simulink model "FingerStrokeAssistance"  (R2016a)
settings: Solver=FixedStepDiscrete  StartTime=0.0  StopTime=inf  FixedStep=.001  RelTol=1e-3
PreLoadFcn:
  | settupFilter;
InitFcn:
  | settupFilter;
  | xpctargetping
values from neighbouring files (symbols this model uses):
  x0low = (eye(size(Alow))-Alow)\Blow*0    [settupFilter.m]
undefined symbols (not defined in the file or in its folder): a_hp, a_lp, Alow, b_hp, b_lp, Blow, Clow, DiscIntNeverNeededParam, Dlow
libraries: simulink x8, slrtlib x8, xpcnilib x4
settings Model: SimulationMode=external  Creator=Admin  LastModifiedBy=Juno
settings SolverCC: EnableConcurrentExecution=on
settings DataIOCC: LimitDataPoints=on  SaveFormat=Array
settings OptimizationCC: BlockReduction=off  OptimizeBlockIOStorage=off  BufferReuse=off  GlobalBufferReuse=off  ExpressionFolding=off  ExpressionDepthLimit=2147483647  LocalBlockOutputs=off
settings DebuggingCC: UnderspecifiedInitializationDetection=Classic  MergeDetectMultiDrivingBlocksExec=none  SolverPrmCheckMsg=warning  StateNameClashWarn=warning
settings HardwareCC: ProdBitPerPointer=32  ProdLargestAtomicFloat=None  ProdWordSize=32  ProdLongLongMode=on  ProdHWDeviceType=Generic->32-bit x86 compatible
settings ModelReferenceCC: PropagateSignalLabelsOutOfModel=off
settings RTWCC: SystemTargetFile=slrt.tlc  TemplateMakefile=slrt_default_tmf  Description=Simulink Real-Time  RTWCompilerOptimization=on
settings ConfigComp: CovModelRefEnable=Off

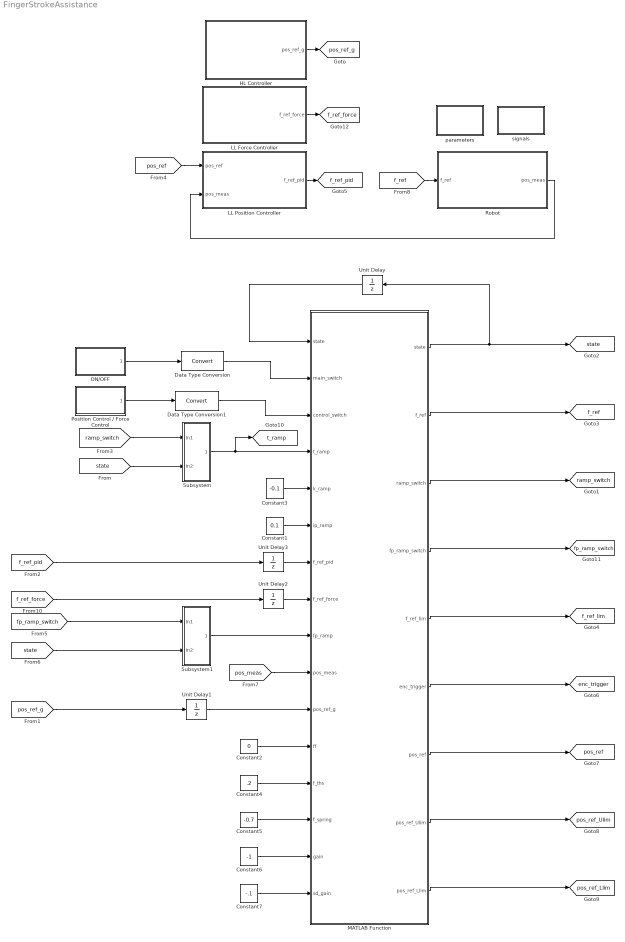
== system FingerStrokeAssistance ==
  Constant1 : Constant  Value=0.1
  Constant2 : Constant  Value=0
  Constant3 : Constant  Value=-0.1
  Constant4 : Constant  Value=.2
  Constant5 : Constant  Value=-0.7
  Constant6 : Constant  Value=-1
  Constant7 : Constant  Value=-.1
  Data Type Conversion : DataTypeConversion
  Data Type Conversion1 : DataTypeConversion
  HL Controller : Subsystem
  LL Force Controller : Subsystem
  LL Position Controller : Subsystem
  MATLAB Function : MATLAB Function  TreatAsAtomicUnit=on
      settings: MinAlgLoopOccurrences=on
  ON/OFF : Subsystem  InitFcn=|  StartFcn=|  StopFcn=|
      InitFcn=|
      | set_param([gcb,'/Constant'],'value','0');                    
      | set_param(gcb,'BackgroundColor',sprintf('[%f,%f,%f]',1,0,0));
      |                                                              
      | set_param(gcb,'MaskDisplay', ['disp(''Not Running'')']);
      StartFcn=|
      | set_param([gcb,'/Constant'],'value','0');                    
      | set_param(gcb,'BackgroundColor',sprintf('[%f,%f,%f]',1,0,0));
      |                                                              
      | set_param(gcb,'MaskDisplay', ['disp(''Not Running'')']);
      StopFcn=|
      | set_param([gcb,'/Constant'],'value','0');                    
      | set_param(gcb,'BackgroundColor',sprintf('[%f,%f,%f]',1,0,0));
      | set_param(gcb,'MaskDisplay', ['disp(''Not Running'')']);
      settings: OpenFcn=|
      | currentState = str2num(get_param([gcb,'/Constant'],'value'));
      | if currentState==1;                                                                       set_param([gcb,'/Constant'],'value','0');
      | set_param(gcb,'BackgroundColor',sprintf('[%f,%f,%f]',1,0,0));                                                   set_param(gcb,'MaskDisplay', ['disp(''Not Running'')']);
      | else                                                                                                                             set_param([gcb,'/Constant'],'value','1');
      | set_param(gcb,'BackgroundColor',sprintf('[%f,%f,%f]',0,1,0));                                            set_param(gcb,'MaskDisplay', ['disp(''Running'')']);
      | 
      | end
      mask Display: disp('Not Running')
  Position Control / Force Control : Subsystem  InitFcn=|  StartFcn=|  StopFcn=|
      InitFcn=|
      | set_param([gcb,'/Constant'],'value','0');                    
      | set_param(gcb,'BackgroundColor',sprintf('[%f,%f,%f]',1,0,0));
      |                                                              
      | set_param(gcb,'MaskDisplay', ['disp(''Not Running'')']);
      StartFcn=|
      | set_param([gcb,'/Constant'],'value','0');                    
      | set_param(gcb,'BackgroundColor',sprintf('[%f,%f,%f]',1,0,0));
      |                                                              
      | set_param(gcb,'MaskDisplay', ['disp(''Not Running'')']);
      StopFcn=|
      | set_param([gcb,'/Constant'],'value','0');                    
      | set_param(gcb,'BackgroundColor',sprintf('[%f,%f,%f]',1,0,0));
      | set_param(gcb,'MaskDisplay', ['disp(''Not Running'')']);
      settings: OpenFcn=|
      | currentState = str2num(get_param([gcb,'/Constant'],'value'));
      | if currentState==1;                                                                       set_param([gcb,'/Constant'],'value','0');
      | set_param(gcb,'BackgroundColor',sprintf('[%f,%f,%f]',1,0,0));                                                   set_param(gcb,'MaskDisplay', ['disp(''Not Running'')']);
      | else                                                                                                                             set_param([gcb,'/Constant'],'value','1');
      | set_param(gcb,'BackgroundColor',sprintf('[%f,%f,%f]',0,1,0));                                            set_param(gcb,'MaskDisplay', ['disp(''Running'')']);
      | 
      | end
      mask Display: disp('Not Running')
  Robot : Subsystem
  Subsystem : Subsystem
  Subsystem1 : Subsystem
  Unit Delay : UnitDelay  InitialCondition=1  SampleTime=-1
  Unit Delay1 : UnitDelay  SampleTime=-1
  Unit Delay2 : UnitDelay  SampleTime=-1
  Unit Delay3 : UnitDelay  SampleTime=-1
  parameters : Subsystem
  signals : Subsystem
  tag scope: enc_trigger=global, f_ref=global, f_ref_force=global, f_ref_lim=global, f_ref_pid=global, fp_ramp_switch=global, pos_ref=global, pos_ref_Llim=global, pos_ref_Ulim=global, pos_ref_g=global, ramp_switch=global, state=global, t_ramp=global
  wires:
  Robot/1(pos_meas) -> LL Position Controller/2(pos_meas)
  MATLAB Function/1(state) -> Unit Delay/1, [state]
  MATLAB Function/2(f_ref) -> [f_ref]
  Constant3/1 -> MATLAB Function/5(k_ramp)
  MATLAB Function/5(f_ref_lim) -> [f_ref_lim]
  MATLAB Function/3(ramp_switch) -> [ramp_switch]
  MATLAB Function/6(enc_trigger) -> [enc_trigger]
  Constant1/1 -> MATLAB Function/6(ip_ramp)
  [f_ref_pid] -> Unit Delay3/1
  MATLAB Function/8(pos_ref_Ulim) -> [pos_ref_Ulim]
  MATLAB Function/9(pos_ref_Llim) -> [pos_ref_Llim]
  [pos_ref] -> LL Position Controller/1(pos_ref)
  MATLAB Function/7(pos_ref) -> [pos_ref]
  Unit Delay3/1 -> MATLAB Function/7(f_ref_pid)
  Subsystem/1(Out1) -> [t_ramp], MATLAB Function/4(t_ramp)
  [ramp_switch] -> Subsystem/1(In1)
  [state] -> Subsystem/2(In2)
  [fp_ramp_switch] -> Subsystem1/1(In1)
  [state] -> Subsystem1/2(In2)
  MATLAB Function/4(fp_ramp_switch) -> [fp_ramp_switch]
  Subsystem1/1(Out1) -> MATLAB Function/9(fp_ramp)
  [pos_meas] -> MATLAB Function/10(pos_meas)
  ON/OFF/1(" ") -> Data Type Conversion/1
  Unit Delay/1 -> MATLAB Function/1("state ")
  [pos_ref_g] -> Unit Delay1/1
  Unit Delay1/1 -> MATLAB Function/11(pos_ref_g)
  LL Position Controller/1(" f_ref_pid") -> [f_ref_pid]
  [f_ref] -> Robot/1(f_ref)
  Data Type Conversion/1 -> MATLAB Function/2(main_switch)
  HL Controller/1(pos_ref_g) -> [pos_ref_g]
  Position Control / Force Control/1(" ") -> Data Type Conversion1/1
  Data Type Conversion1/1 -> MATLAB Function/3(control_switch)
  [f_ref_force] -> Unit Delay2/1
  Unit Delay2/1 -> MATLAB Function/8(f_ref_force)
  LL Force Controller/1(" f_ref_force") -> [f_ref_force]
  Constant2/1 -> MATLAB Function/12(ff)
  Constant5/1 -> MATLAB Function/14(f_spring)
  Constant6/1 -> MATLAB Function/15(gain)
  Constant4/1 -> MATLAB Function/13(f_ths)
  Constant7/1 -> MATLAB Function/16(sd_gain)

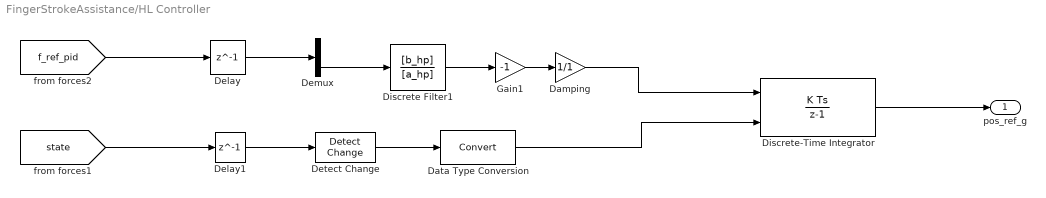
== system FingerStrokeAssistance/HL Controller ==
  Damping : Gain  Gain=1/1
  Data Type Conversion : DataTypeConversion
  Delay : Delay  DelayLength=1  InitialCondition=0
  Delay1 : Delay  DelayLength=1  InitialCondition=0
  Demux : Demux  Outputs=2
  Detect Change : simulink/Logic and Bit Operations/Detect Change  vinit=0  OutDataTypeStr=boolean
  Discrete Filter1 : DiscreteFilter  Numerator=[b_hp]  Denominator=[a_hp]
  Discrete-Time Integrator : DiscreteIntegrator  ExternalReset=either  InitialConditionSetting=State (most efficient)  SampleTime=-1  LimitOutput=on  UpperSaturationLimit=1  LowerSaturationLimit=0  ICPrevOutput=DiscIntNeverNeededParam  ICPrevScaledInput=DiscIntNeverNeededParam
  Gain1 : Gain  Gain=-1
  pos_ref_g : Outport
  wires:
  [f_ref_pid] -> Delay/1
  [state] -> Delay1/1
  Discrete-Time Integrator/1 -> pos_ref_g/1
  Detect Change/1 -> Data Type Conversion/1
  Delay1/1 -> Detect Change/1
  Delay/1 -> Demux/1
  Data Type Conversion/1 -> Discrete-Time Integrator/2
  Gain1/1 -> Damping/1
  Damping/1 -> Discrete-Time Integrator/1
  Demux/2 -> Discrete Filter1/1
  Discrete Filter1/1 -> Gain1/1

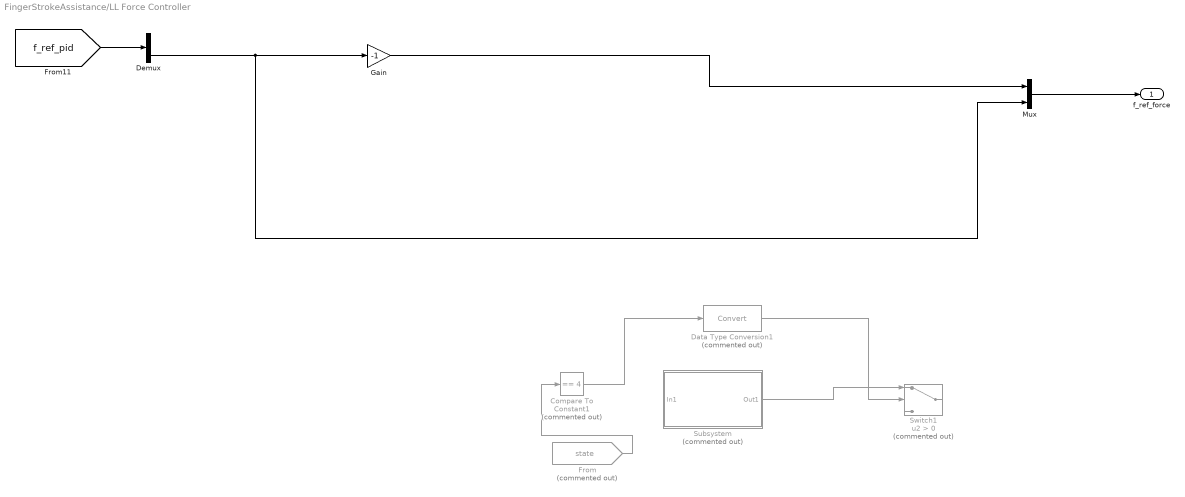
== system FingerStrokeAssistance/LL Force Controller ==
  Compare To Constant1 : simulink/Logic and Bit Operations/Compare To Constant  Commented=on  relop===  const=4  OutDataTypeStr=boolean
  Data Type Conversion1 : DataTypeConversion  Commented=on
  Demux : Demux  Outputs=2
  From : From  Commented=on  GotoTag=state  TagVisibility=global
  Gain : Gain  Gain=-1
  Mux : Mux  Inputs=2
  Subsystem : Subsystem  Commented=on
  Switch1 : Switch  Commented=on  Criteria=u2 > Threshold
  " f_ref_force" : Outport
  wires:
  [f_ref_pid] -> Demux/1
  Demux/2 -> Mux/2, Gain/1
  Subsystem/1(Out1) -> Switch1/1
  Data Type Conversion1/1 -> Switch1/2
  From/1 -> Compare To Constant1/1
  Compare To Constant1/1 -> Data Type Conversion1/1
  Mux/1 -> " f_ref_force"/1
  Gain/1 -> Mux/1

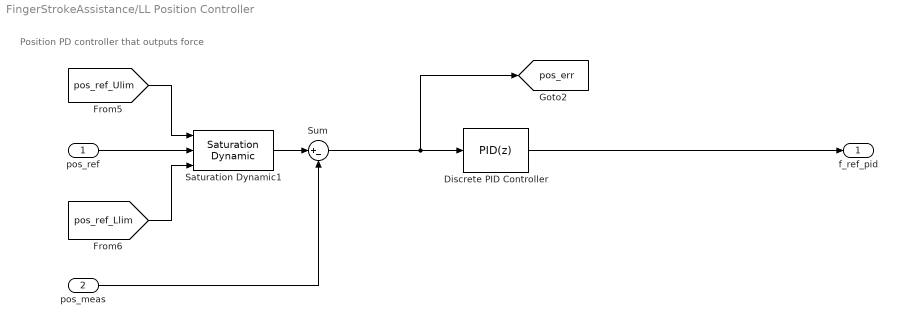
== system FingerStrokeAssistance/LL Position Controller ==
  note: Position PD controller that outputs force
  pos_ref : Inport
  pos_meas : Inport  Port=2
  Discrete PID Controller : simulink/Continuous/PID Controller  Controller=PID  TimeDomain=Discrete-time  SampleTime=-1  IntegratorMethod=Forward Euler  FilterMethod=Forward Euler  Form=Parallel  UseFilter=on  ControllerParametersSource=internal  P=10  I=0  D=0  N=100  InitialConditionSource=internal  InitialConditionForIntegrator=0  InitialConditionForFilter=0  ExternalReset=none  LimitOutput=off  UpperSaturationLimit=inf  LowerSaturationLimit=-inf  LinearizeAsGain=off  AntiWindupMode=none  Kb=1  TrackingMode=off  Kt=1  PParamMin=[]  PParamMax=[]  IParamMin=[]  IParamMax=[]  DParamMin=[]  DParamMax=[]  NParamMin=[]  NParamMax=[]  KbParamMin=[]  KbParamMax=[]  KtParamMin=[]  KtParamMax=[]  POutMin=[]  POutMax=[]  IOutMin=[]  IOutMax=[]  DOutMin=[]  DOutMax=[]  NOutMin=[]  NOutMax=[]  KbOutMin=[]  KbOutMax=[]  KtOutMin=[]  KtOutMax=[]  IntegratorOutMin=[]  IntegratorOutMax=[]  FilterOutMin=[]  FilterOutMax=[]  SumOutMin=[]  SumOutMax=[]  SumI1OutMin=[]  SumI1OutMax=[]  SumI2OutMin=[]  SumI2OutMax=[]  SumI3OutMin=[]  SumI3OutMax=[]  SumDOutMin=[]  SumDOutMax=[]  SaturationOutMin=[]  SaturationOutMax=[]  IntegratorContinuousStateAttributes=''  IntegratorStateMustResolveToSignalObject=off  IntegratorRTWStateStorageClass=Auto  FilterContinuousStateAttributes=''  FilterStateMustResolveToSignalObject=off  FilterRTWStateStorageClass=Auto  DifferentiatorICPrevScaledInput=0  DifferentiatorOutMin=[]  DifferentiatorOutMax=[]
  Saturation Dynamic1 : simulink/Discontinuities/Saturation Dynamic  OutMin=[]  OutMax=[]  OutDataTypeStr=Inherit: Same as second input  OutDataType=fixdt(1, 16)  OutScaling=2^-10  DoSatur=off
  Sum : Sum  Inputs=|+-
  " f_ref_pid" : Outport
  tag scope: pos_err=global
  wires:
  pos_meas/1 -> Sum/2
  Sum/1 -> Discrete PID Controller/1, [pos_err]
  Saturation Dynamic1/1 -> Sum/1
  pos_ref/1 -> Saturation Dynamic1/2
  [pos_ref_Ulim] -> Saturation Dynamic1/1
  [pos_ref_Llim] -> Saturation Dynamic1/3
  Discrete PID Controller/1 -> " f_ref_pid"/1

== system FingerStrokeAssistance/ON//OFF ==
  note: ON/OFF
  Constant : Constant  Value=0  OutDataTypeStr=boolean
  " " : Outport
  wires:
  Constant/1 -> " "/1

== system FingerStrokeAssistance/Position Control // Force Control ==
  note: ON/OFF
  Constant : Constant  Value=0  OutDataTypeStr=boolean
  " " : Outport
  wires:
  Constant/1 -> " "/1

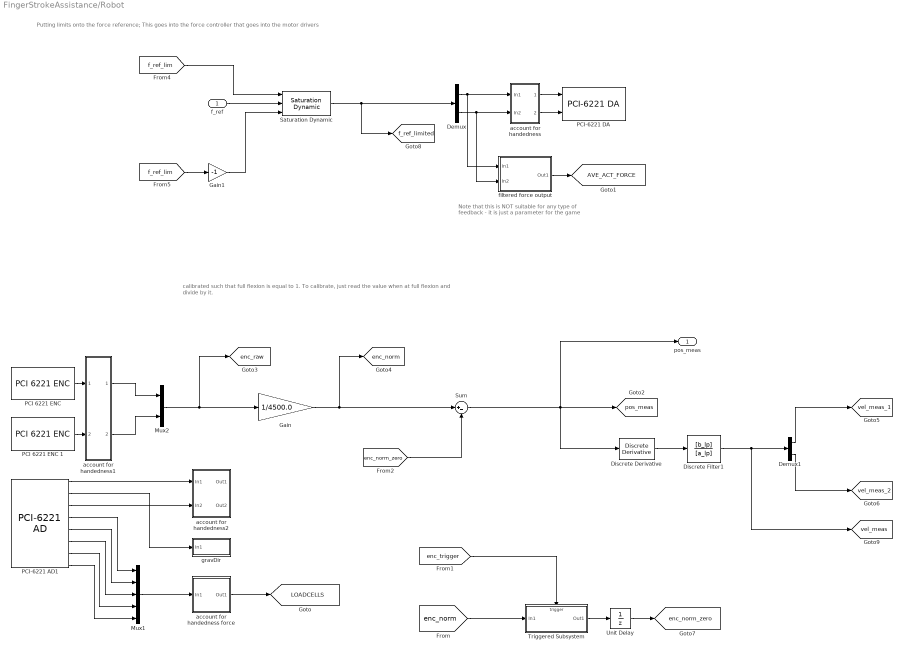
== system FingerStrokeAssistance/Robot ==
  note: Note that this is NOT suitable for any type
      | of feedback - it is just a parameter for the game
  note: calibrated such that full flexion is equal to 1. To calibrate, just read the value when at full flexion and divide by it.
  note: Putting limits onto the force reference; This goes into the force controller that goes into the motor drivers
  f_ref : Inport
  Demux : Demux  Outputs=2
  Demux1 : Demux  Outputs=2
  Discrete Derivative : simulink/Discrete/Discrete Derivative  gainval=1.0  ICPrevScaledInput=0.0  OutMin=[]  OutMax=[]  OutDataType=fixdt(1, 16)  OutScaling=2^-10  DoSatur=off
  Discrete Filter1 : DiscreteFilter  Numerator=[b_lp]  Denominator=[a_lp]
  Gain : Gain  Gain=1/4500.0
  Gain1 : Gain  Gain=-1
  Mux1 : Mux  Inputs=5
  Mux2 : Mux  Inputs=2
  "PCI 6221 ENC " : xpcnilib/Incremental Encoder/PCI 6221 ENC   channel=0  countMode=Quadrature Mode x4  initCount=0  reload=off  indexPhase=A low B low  filter=Minimum pulse width 125 nanoseconds  sampleTime=0.001  slot=-1
  PCI 6221 ENC 1 : xpcnilib/Incremental Encoder/PCI 6221 ENC   channel=1  countMode=Quadrature Mode x4  initCount=0  reload=off  indexPhase=A low B low  filter=Minimum pulse width 125 nanoseconds  sampleTime=0.001  slot=-1
  PCI-6221 AD1 : xpcnilib/A//D/M Series/PCI-6221 AD  channel=[1 2 3 4 5 6 7 8]  range=[10]  coupling=[0]  scantime=5e-6  sampletime=0.001  slot=-1
  PCI-6221 DA : xpcnilib/D//A/M Series/PCI-6221 DA  channel=[1 2]  reset=[1]  initValue=[0]  sampletime=0.001  slot=-1
  Saturation Dynamic : simulink/Discontinuities/Saturation Dynamic  OutMin=[]  OutMax=[]  OutDataTypeStr=Inherit: Same as second input  OutDataType=fixdt(1, 16)  OutScaling=2^-10  DoSatur=off
  Sum : Sum  Inputs=|+-
  Triggered Subsystem : Subsystem  TreatAsAtomicUnit=on
  Unit Delay : UnitDelay  SampleTime=-1
  account for handedness : Subsystem
  account for handedness force : Subsystem
  account for handedness1 : Subsystem
  account for handedness2 : Subsystem
  filtered force output : Subsystem
  gravDir : Subsystem
  pos_meas : Outport
  tag scope: AVE_ACT_FORCE=global, LOADCELLS=global, enc_norm=global, enc_norm_zero=global, enc_raw=global, f_ref_limited=global, pos_meas=global, vel_meas=global, vel_meas_1=global, vel_meas_2=global
  wires:
  Demux/1 -> filtered force output/1(In1), account for handedness/1(In1)
  Demux/2 -> filtered force output/2(In2), account for handedness/2(In2)
  account for handedness/2(Out2) -> PCI-6221 DA/2
  account for handedness/1(Out1) -> PCI-6221 DA/1
  "PCI 6221 ENC "/1 -> account for handedness1/1(In1)
  PCI 6221 ENC 1/1 -> account for handedness1/2(In2)
  PCI-6221 AD1/1 -> account for handedness2/1(In1)
  PCI-6221 AD1/3 -> account for handedness2/2(In2)
  PCI-6221 AD1/4 -> Mux1/1
  PCI-6221 AD1/5 -> Mux1/2
  PCI-6221 AD1/6 -> Mux1/3
  PCI-6221 AD1/7 -> Mux1/4
  PCI-6221 AD1/8 -> Mux1/5
  Mux1/1 -> account for handedness force/1(In1)
  account for handedness force/1(Out1) -> [LOADCELLS]
  PCI-6221 AD1/2 -> gravDir/1(In1)
  filtered force output/1(Out1) -> [AVE_ACT_FORCE]
  account for handedness1/1(Out1) -> Mux2/1
  account for handedness1/2(Out2) -> Mux2/2
  Mux2/1 -> [enc_raw], Gain/1
  Demux1/1 -> [vel_meas_1]
  Demux1/2 -> [vel_meas_2]
  Gain/1 -> Sum/1, [enc_norm]
  [enc_norm] -> Triggered Subsystem/1(In1)
  Triggered Subsystem/1(Out1) -> Unit Delay/1
  [enc_norm_zero] -> Sum/2
  Unit Delay/1 -> [enc_norm_zero]
  Sum/1 -> [pos_meas], pos_meas/1, Discrete Derivative/1
  [enc_trigger] -> Triggered Subsystem/Trigger
  Saturation Dynamic/1 -> [f_ref_limited], Demux/1
  Gain1/1 -> Saturation Dynamic/3
  [f_ref_lim] -> Saturation Dynamic/1
  [f_ref_lim] -> Gain1/1
  f_ref/1 -> Saturation Dynamic/2
  Discrete Derivative/1 -> Discrete Filter1/1
  Discrete Filter1/1 -> [vel_meas], Demux1/1

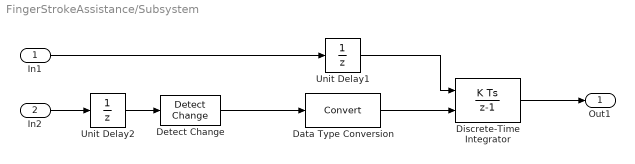
== system FingerStrokeAssistance/Subsystem ==
  In1 : Inport
  In2 : Inport  Port=2
  Data Type Conversion : DataTypeConversion
  Detect Change : simulink/Logic and Bit Operations/Detect Change  vinit=0  OutDataTypeStr=boolean
  Discrete-Time Integrator : DiscreteIntegrator  ExternalReset=either  InitialConditionSetting=State (most efficient)  SampleTime=-1  UpperSaturationLimit=0.9  LowerSaturationLimit=0  ICPrevOutput=DiscIntNeverNeededParam  ICPrevScaledInput=DiscIntNeverNeededParam
  Unit Delay1 : UnitDelay  SampleTime=-1
  Unit Delay2 : UnitDelay  SampleTime=-1
  Out1 : Outport
  wires:
  In1/1 -> Unit Delay1/1
  Unit Delay1/1 -> Discrete-Time Integrator/1
  Discrete-Time Integrator/1 -> Out1/1
  In2/1 -> Unit Delay2/1
  Data Type Conversion/1 -> Discrete-Time Integrator/2
  Detect Change/1 -> Data Type Conversion/1
  Unit Delay2/1 -> Detect Change/1

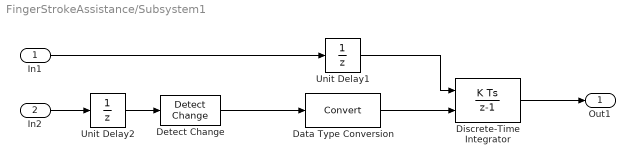
== system FingerStrokeAssistance/Subsystem1 ==
  In1 : Inport
  In2 : Inport  Port=2
  Data Type Conversion : DataTypeConversion
  Detect Change : simulink/Logic and Bit Operations/Detect Change  vinit=0  OutDataTypeStr=boolean
  Discrete-Time Integrator : DiscreteIntegrator  ExternalReset=either  InitialConditionSetting=State (most efficient)  SampleTime=-1  UpperSaturationLimit=0.9  LowerSaturationLimit=0  ICPrevOutput=DiscIntNeverNeededParam  ICPrevScaledInput=DiscIntNeverNeededParam
  Unit Delay1 : UnitDelay  SampleTime=-1
  Unit Delay2 : UnitDelay  SampleTime=-1
  Out1 : Outport
  wires:
  Unit Delay2/1 -> Detect Change/1
  Detect Change/1 -> Data Type Conversion/1
  Data Type Conversion/1 -> Discrete-Time Integrator/2
  In2/1 -> Unit Delay2/1
  Discrete-Time Integrator/1 -> Out1/1
  Unit Delay1/1 -> Discrete-Time Integrator/1
  In1/1 -> Unit Delay1/1

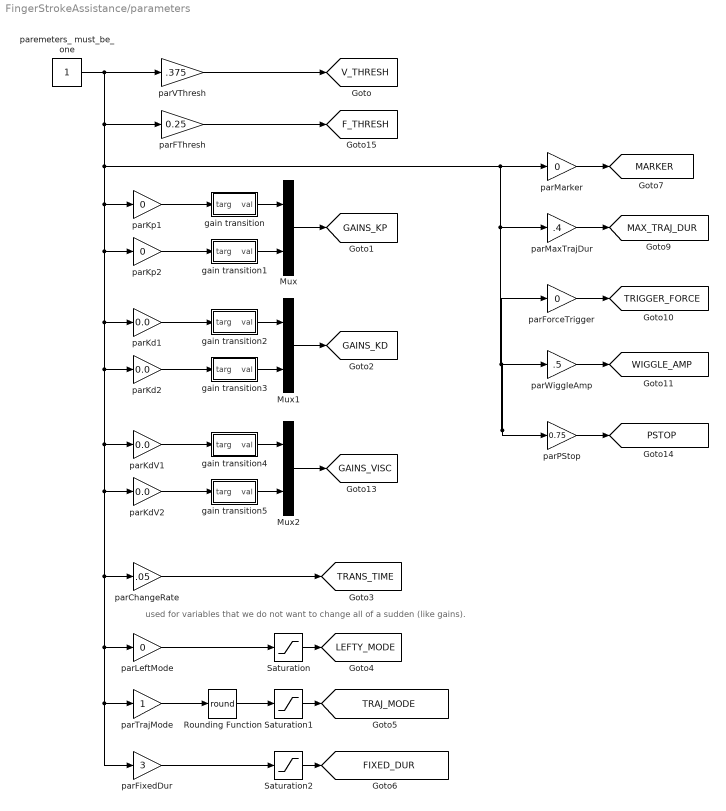
== system FingerStrokeAssistance/parameters ==
  note: used for variables that we do not want to change all of a sudden (like gains).
  Mux : Mux  Inputs=2
  Mux1 : Mux  Inputs=2
  Mux2 : Mux  Inputs=2
  Rounding Function : Rounding  Operator=round
  Saturation : Saturate  UpperLimit=1  LowerLimit=0
  Saturation1 : Saturate  UpperLimit=4  LowerLimit=1
  Saturation2 : Saturate  UpperLimit=10  LowerLimit=.25
  gain transition : Subsystem
  gain transition1 : Subsystem
  gain transition2 : Subsystem
  gain transition3 : Subsystem
  gain transition4 : Subsystem
  gain transition5 : Subsystem
  parChangeRate : Gain  Gain=.05
  parFThresh : Gain  Gain=0.25
  parFixedDur : Gain  Gain=3
  parForceTrigger : Gain  Gain=0
  parKd1 : Gain  Gain=0.0
  parKd2 : Gain  Gain=0.0
  parKdV1 : Gain  Gain=0.0
  parKdV2 : Gain  Gain=0.0
  parKp1 : Gain  Gain=0
  parKp2 : Gain  Gain=0
  parLeftMode : Gain  Gain=0
  parMarker : Gain  Gain=0
  parMaxTrajDur : Gain  Gain=.4
  parPStop : Gain  Gain=0.75
  parTrajMode : Gain
  parVThresh : Gain  Gain=.375
  parWiggleAmp : Gain  Gain=.5
  paremeters_ must_be_one : Constant
  tag scope: FIXED_DUR=global, F_THRESH=global, GAINS_KD=global, GAINS_KP=global, GAINS_VISC=global, LEFTY_MODE=global, MARKER=global, MAX_TRAJ_DUR=global, PSTOP=global, TRAJ_MODE=global, TRANS_TIME=global, TRIGGER_FORCE=global, V_THRESH=global, WIGGLE_AMP=global
  wires:
  Mux/1 -> [GAINS_KP]
  Mux1/1 -> [GAINS_KD]
  Saturation/1 -> [LEFTY_MODE]
  gain transition/1(val) -> Mux/1
  gain transition1/1(val) -> Mux/2
  gain transition2/1(val) -> Mux1/1
  gain transition3/1(val) -> Mux1/2
  parVThresh/1 -> [V_THRESH]
  parKp1/1 -> gain transition/1(targ)
  parKp2/1 -> gain transition1/1(targ)
  parKd1/1 -> gain transition2/1(targ)
  parKd2/1 -> gain transition3/1(targ)
  parChangeRate/1 -> [TRANS_TIME]
  parLeftMode/1 -> Saturation/1
  Saturation1/1 -> [TRAJ_MODE]
  parTrajMode/1 -> Rounding Function/1
  Saturation2/1 -> [FIXED_DUR]
  parFixedDur/1 -> Saturation2/1
  Rounding Function/1 -> Saturation1/1
  parMarker/1 -> [MARKER]
  parMaxTrajDur/1 -> [MAX_TRAJ_DUR]
  parForceTrigger/1 -> [TRIGGER_FORCE]
  parWiggleAmp/1 -> [WIGGLE_AMP]
  Mux2/1 -> [GAINS_VISC]
  gain transition4/1(val) -> Mux2/1
  gain transition5/1(val) -> Mux2/2
  parKdV1/1 -> gain transition4/1(targ)
  parKdV2/1 -> gain transition5/1(targ)
  paremeters_ must_be_one/1 -> parVThresh/1, parFThresh/1, parKp1/1, parKp2/1, parKd1/1, parKd2/1, parKdV1/1, parKdV2/1, parChangeRate/1, parLeftMode/1, parFixedDur/1, parTrajMode/1, parPStop/1, parWiggleAmp/1, parForceTrigger/1, parMaxTrajDur/1, parMarker/1
  parPStop/1 -> [PSTOP]
  parFThresh/1 -> [F_THRESH]

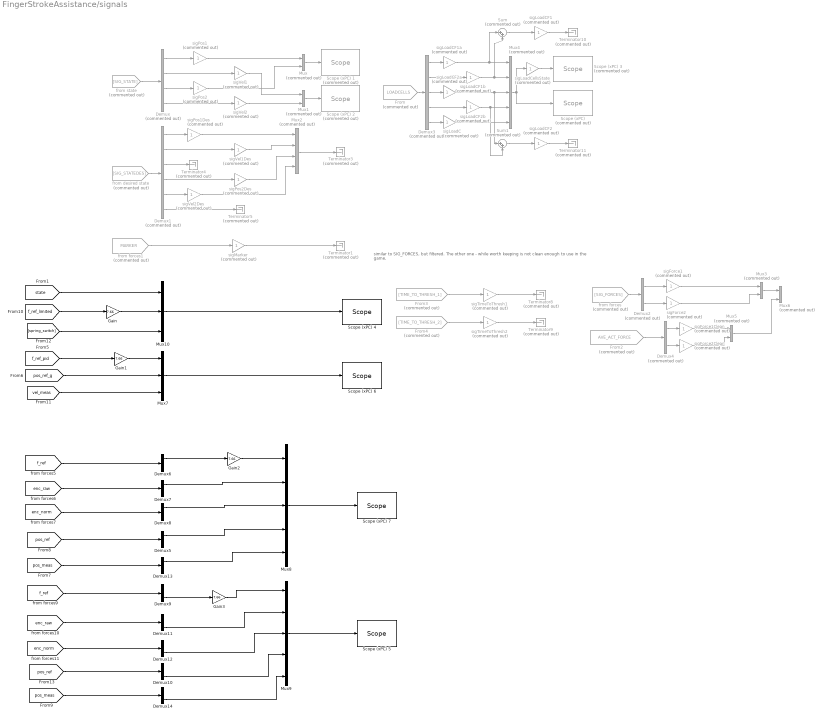
== system FingerStrokeAssistance/signals ==
  note: similar to SIG_FORCES, but filtered. The other one - while worth keeping is not clean enough to use in the game.
  Demux : Demux  Commented=on
  Demux1 : Demux  Commented=on  Outputs=6
  Demux{5..14} (10 alike) : Demux  Outputs=2
  Demux2 : Demux  Commented=on  Outputs=2
  Demux3 : Demux  Commented=on  Outputs=5
  Demux4 : Demux  Commented=on  Outputs=2
  From : From  Commented=on  GotoTag=LOADCELLS  TagVisibility=global
  From2 : From  Commented=on  GotoTag=AVE_ACT_FORCE  TagVisibility=global
  From3 : From  Commented=on  GotoTag=TIME_TO_THRESH_1
  From4 : From  Commented=on  GotoTag=TIME_TO_THRESH_2
  Gain{,1..3} (4 alike) : Gain  Gain=7.66
  Mux{,1,3,5..6} (5 alike) : Mux  Commented=on  Inputs=2
  Mux10 : Mux  Inputs=3
  Mux2 : Mux  Commented=on
  Mux4 : Mux  Commented=on  Inputs=5
  Mux7 : Mux  Inputs=3
  Mux8 : Mux  Inputs=5
  Mux9 : Mux  Inputs=5
  "Scope (xPC) " : slrtlib/Displays and Logging/Scope   Commented=on  scopeno=5  scopetype=Target  autostart=on  viewmode=Graphical redraw  formatstr='%15.6f'  grid=on  ylimits=[-3,3]  nosamples=500  noprepostsamples=0  interleave=1  triggermode=FreeRun  triggersignal=1  trigsignalfromport=off  triggerlevel=0.0  triggerslope=Either  triggerscope=1  triggersample=0  filename=data.dat  mode=Lazy  writesize=512  autorestart=off  dynamicfilemode=off  maxwritefilesize=512*1024^2
  Scope (xPC) 1 : slrtlib/Displays and Logging/Scope   Commented=on  scopeno=1  scopetype=Target  autostart=on  viewmode=Graphical redraw  formatstr='%15.6f'  grid=on  ylimits=[0,1.1]  nosamples=500  noprepostsamples=0  interleave=1  triggermode=FreeRun  triggersignal=1  trigsignalfromport=off  triggerlevel=0.0  triggerslope=Either  triggerscope=1  triggersample=0  filename=data.dat  mode=Lazy  writesize=512  autorestart=off  dynamicfilemode=off  maxwritefilesize=512*1024^2
  Scope (xPC) 2 : slrtlib/Displays and Logging/Scope   Commented=on  scopeno=2  scopetype=Target  autostart=on  viewmode=Graphical redraw  formatstr='%15.6f'  grid=on  ylimits=[-10,10]  nosamples=500  noprepostsamples=0  interleave=1  triggermode=FreeRun  triggersignal=1  trigsignalfromport=off  triggerlevel=0.0  triggerslope=Either  triggerscope=1  triggersample=0  filename=data.dat  mode=Lazy  writesize=512  autorestart=off  dynamicfilemode=off  maxwritefilesize=512*1024^2
  Scope (xPC) 3 : slrtlib/Displays and Logging/Scope   Commented=on  scopeno=4  scopetype=File  autostart=on  viewmode=Graphical redraw  formatstr='%15.6f'  grid=on  ylimits=[0,0]  nosamples=5000  noprepostsamples=0  interleave=1  triggermode=FreeRun  triggersignal=1  trigsignalfromport=off  triggerlevel=0.0  triggerslope=Either  triggerscope=1  triggersample=0  filename=fLogData.dat  mode=Lazy  writesize=512  autorestart=off  dynamicfilemode=off  maxwritefilesize=512*1024^2
  Scope (xPC) 4 : slrtlib/Displays and Logging/Scope   scopeno=1  scopetype=Target  autostart=on  viewmode=Numerical  formatstr='state:%15.6f,f_ref_limited_1:%15.6f,f_ref_limited_2:%15.6f,vel_meas_1:%15.6f,vel_meas_2:%15.6f'  grid=on  ylimits=[-1,5]  nosamples=10  noprepostsamples=0  interleave=1  triggermode=FreeRun  triggersignal=1  trigsignalfromport=off  triggerlevel=0.0  triggerslope=Either  triggerscope=1  triggersample=0  filename=data.dat  mode=Lazy  writesize=512  autorestart=off  dynamicfilemode=off  maxwritefilesize=512*1024^2
  Scope (xPC) 5 : slrtlib/Displays and Logging/Scope   scopeno=4  scopetype=Target  autostart=on  viewmode=Numerical  formatstr='f_ref2:%15.6f,enc_raw2:%15.6f,enc_norm2:%15.6f,pos_ref_2:%15.6f,pos_meas_2:%15.6f'  grid=on  ylimits=[.03,.1]  nosamples=10  noprepostsamples=0  interleave=1  triggermode=FreeRun  triggersignal=1  trigsignalfromport=off  triggerlevel=0.0  triggerslope=Either  triggerscope=1  triggersample=0  filename=data.dat  mode=Lazy  writesize=512  autorestart=off  dynamicfilemode=off  maxwritefilesize=512*1024^2
  Scope (xPC) 6 : slrtlib/Displays and Logging/Scope   scopeno=2  scopetype=Target  autostart=on  viewmode=Numerical  formatstr='f_ref_pid_1:%15.6f,f_ref_pid_2:%15.6f,pos_ref_g:%15.6f,vel_meas_1:%15.6f,vel_meas_2:%15.6f'  grid=on  ylimits=[-2.5,2.5]  nosamples=10  noprepostsamples=0  interleave=1  triggermode=FreeRun  triggersignal=1  trigsignalfromport=off  triggerlevel=0.0  triggerslope=Either  triggerscope=1  triggersample=0  filename=data.dat  mode=Lazy  writesize=512  autorestart=off  dynamicfilemode=off  maxwritefilesize=512*1024^2
  Scope (xPC) 7 : slrtlib/Displays and Logging/Scope   scopeno=3  scopetype=Target  autostart=on  viewmode=Numerical  formatstr='f_ref1:%15.6f N,enc_raw:%15.6f,enc_norm:%15.6f,pos_ref_1:%15.6f,pos_meas_1:%15.6f'  grid=on  ylimits=[.03,.1]  nosamples=10  noprepostsamples=0  interleave=1  triggermode=FreeRun  triggersignal=1  trigsignalfromport=off  triggerlevel=0.0  triggerslope=Either  triggerscope=1  triggersample=0  filename=data.dat  mode=Lazy  writesize=512  autorestart=off  dynamicfilemode=off  maxwritefilesize=512*1024^2
  Sum : Sum  Commented=on  Inputs=|++
  Sum1 : Sum  Commented=on  Inputs=|++
  Terminator{1,3..5,8..11} (8 alike) : Terminator  Commented=on
  from desired state : From  Commented=on  GotoTag=SIG_STATEDES
  from forces : From  Commented=on  GotoTag=SIG_FORCES  TagVisibility=global
  from forces1 : From  Commented=on  GotoTag=MARKER  TagVisibility=global
  from state : From  Commented=on  GotoTag=SIG_STATE  TagVisibility=global
  sigForce1 : Gain  Commented=on
  sigForce1Clean : Gain  Commented=on
  sigForce2 : Gain  Commented=on
  sigForce2Clean : Gain  Commented=on
  sigLoadC : Gain  Commented=on
  sigLoadCF1 : Gain  Commented=on
  sigLoadCF1a : Gain  Commented=on
  sigLoadCF1b : Gain  Commented=on
  sigLoadCF2 : Gain  Commented=on
  sigLoadCF2a : Gain  Commented=on
  sigLoadCF2b : Gain  Commented=on
  sigLoadCellsState : Gain  Commented=on
  sigMarker : Gain  Commented=on
  sigPos1 : Gain  Commented=on
  sigPos1Des : Gain  Commented=on
  sigPos2 : Gain  Commented=on
  sigPos2Des : Gain  Commented=on
  sigTimeToThresh1 : Gain  Commented=on
  sigTimeToThresh2 : Gain  Commented=on
  sigVel1 : Gain  Commented=on
  sigVel1Des : Gain  Commented=on
  sigVel2 : Gain  Commented=on
  sigVel2Des : Gain  Commented=on
  wires:
  from state/1 -> Demux/1
  Demux/1 -> sigPos1/1
  Demux/2 -> sigVel1/1
  Demux/3 -> sigPos2/1
  Demux/4 -> sigVel2/1
  from desired state/1 -> Demux1/1
  Demux1/1 -> sigPos1Des/1
  Demux1/2 -> sigVel1Des/1
  Demux1/3 -> Terminator4/1
  Demux1/4 -> sigPos2Des/1
  Demux1/5 -> sigVel2Des/1
  Demux1/6 -> Terminator5/1
  Mux/1 -> Scope (xPC) 1/1
  Mux1/1 -> Scope (xPC) 2/1
  sigPos1/1 -> Mux/1
  sigPos2/1 -> Mux/2
  sigVel1/1 -> Mux1/1
  sigVel2/1 -> Mux1/2
  sigPos1Des/1 -> Mux2/1
  sigVel1Des/1 -> Mux2/2
  sigPos2Des/1 -> Mux2/3
  sigVel2Des/1 -> Mux2/4
  Mux2/1 -> Terminator3/1
  from forces/1 -> Demux2/1
  Demux2/1 -> sigForce1/1
  Demux2/2 -> sigForce2/1
  sigForce1/1 -> Mux3/1
  sigForce2/1 -> Mux3/2
  from forces1/1 -> sigMarker/1
  sigMarker/1 -> Terminator1/1
  From/1 -> Demux3/1
  Demux3/1 -> sigLoadCF1a/1
  Demux3/2 -> sigLoadCF1b/1
  Demux3/3 -> sigLoadCF2a/1
  Demux3/4 -> sigLoadCF2b/1
  Demux3/5 -> sigLoadC/1
  sigLoadCF1a/1 -> Sum/1, Mux4/1
  sigLoadCF1b/1 -> Sum/2, Mux4/2
  sigLoadCF2a/1 -> Sum1/1, Mux4/3
  sigLoadCF2b/1 -> Mux4/4, Sum1/2
  sigLoadC/1 -> Mux4/5
  Mux4/1 -> sigLoadCellsState/1, "Scope (xPC) "/1
  From2/1 -> Demux4/1
  Demux4/1 -> sigForce1Clean/1
  Demux4/2 -> sigForce2Clean/1
  sigForce1Clean/1 -> Mux5/1
  sigForce2Clean/1 -> Mux5/2
  sigTimeToThresh1/1 -> Terminator8/1
  From3/1 -> sigTimeToThresh1/1
  sigTimeToThresh2/1 -> Terminator9/1
  From4/1 -> sigTimeToThresh2/1
  sigLoadCellsState/1 -> Scope (xPC) 3/1
  Sum/1 -> sigLoadCF1/1
  Sum1/1 -> sigLoadCF2/1
  sigLoadCF1/1 -> Terminator10/1
  sigLoadCF2/1 -> Terminator11/1
  Mux3/1 -> Mux6/1
  Mux5/1 -> Mux6/2
  Mux10/1 -> Scope (xPC) 4/1
  Mux8/1 -> Scope (xPC) 7/1
  [enc_raw] -> Demux7/1
  Demux7/1 -> Mux8/2
  [enc_norm] -> Demux8/1
  Demux8/1 -> Mux8/3
  [pos_ref] -> Demux5/1
  Mux9/1 -> Scope (xPC) 5/1
  [enc_raw] -> Demux11/1
  [enc_norm] -> Demux12/1
  [pos_ref] -> Demux10/1
  Demux10/2 -> Mux9/4
  Demux11/2 -> Mux9/2
  Demux12/2 -> Mux9/3
  Demux5/1 -> Mux8/4
  [state] -> Mux10/1
  [f_ref] -> Demux6/1
  Demux6/1 -> Gain2/1
  [f_ref] -> Demux9/1
  Demux9/2 -> Gain3/1
  Mux7/1 -> Scope (xPC) 6/1
  [pos_ref_g] -> Mux7/2
  [pos_meas] -> Demux13/1
  Demux13/1 -> Mux8/5
  [pos_meas] -> Demux14/1
  Demux14/2 -> Mux9/5
  [f_ref_limited] -> Gain/1
  [vel_meas] -> Mux7/3
  [spring_switch] -> Mux10/3
  Gain/1 -> Mux10/2
  [f_ref_pid] -> Gain1/1
  Gain2/1 -> Mux8/1
  Gain3/1 -> Mux9/1
  Gain1/1 -> Mux7/1

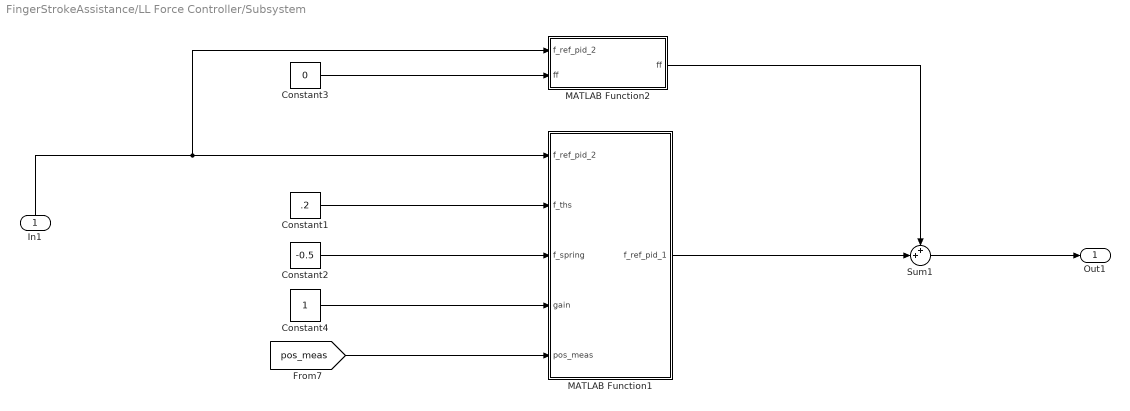
== system FingerStrokeAssistance/LL Force Controller/Subsystem ==
  In1 : Inport
  Constant1 : Constant  Value=.2
  Constant2 : Constant  Value=-0.5
  Constant3 : Constant  Value=0
  Constant4 : Constant
  MATLAB Function1 : MATLAB Function  TreatAsAtomicUnit=on
  MATLAB Function2 : MATLAB Function  TreatAsAtomicUnit=on
  Sum1 : Sum  Inputs=++|
  Out1 : Outport
  wires:
  Constant2/1 -> MATLAB Function1/3(f_spring)
  Constant4/1 -> MATLAB Function1/4(gain)
  MATLAB Function1/1(f_ref_pid_1) -> Sum1/2
  Constant3/1 -> MATLAB Function2/2("ff ")
  MATLAB Function2/1(ff) -> Sum1/1
  Constant1/1 -> MATLAB Function1/2(f_ths)
  In1/1 -> MATLAB Function2/1(f_ref_pid_2), MATLAB Function1/1(f_ref_pid_2)
  Sum1/1 -> Out1/1
  [pos_meas] -> MATLAB Function1/5(pos_meas)

== system FingerStrokeAssistance/Robot/Triggered Subsystem ==
  In1 : Inport
  Trigger : TriggerPort  VariantControl=Variant
  Out1 : Outport  InitialOutput=[0]
  wires:
  In1/1 -> Out1/1

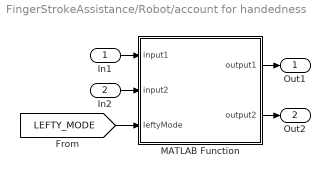
== system FingerStrokeAssistance/Robot/account for handedness ==
  In1 : Inport
  In2 : Inport  Port=2
  MATLAB Function : MATLAB Function  TreatAsAtomicUnit=on
  Out1 : Outport
  Out2 : Outport  Port=2
  wires:
  MATLAB Function/1(output1) -> Out1/1
  MATLAB Function/2(output2) -> Out2/1
  In1/1 -> MATLAB Function/1(input1)
  In2/1 -> MATLAB Function/2(input2)
  [LEFTY_MODE] -> MATLAB Function/3(leftyMode)

== system FingerStrokeAssistance/Robot/account for handedness force ==
  In1 : Inport
  MATLAB Function : MATLAB Function  TreatAsAtomicUnit=on
  Out1 : Outport
  wires:
  [LEFTY_MODE] -> MATLAB Function/2(leftyMode)
  MATLAB Function/1(output) -> Out1/1
  In1/1 -> MATLAB Function/1(inp1)

== system FingerStrokeAssistance/Robot/account for handedness1 ==
  In1 : Inport
  In2 : Inport  Port=2
  MATLAB Function : MATLAB Function  TreatAsAtomicUnit=on
  Out1 : Outport
  Out2 : Outport  Port=2
  wires:
  MATLAB Function/1(output1) -> Out1/1
  MATLAB Function/2(output2) -> Out2/1
  In1/1 -> MATLAB Function/1(input1)
  In2/1 -> MATLAB Function/2(input2)
  [LEFTY_MODE] -> MATLAB Function/3(leftyMode)

== system FingerStrokeAssistance/Robot/account for handedness2 ==
  In1 : Inport
  In2 : Inport  Port=2
  MATLAB Function : MATLAB Function  TreatAsAtomicUnit=on
  Out1 : Outport
  Out2 : Outport  Port=2
  wires:
  MATLAB Function/1(output1) -> Out1/1
  MATLAB Function/2(output2) -> Out2/1
  In1/1 -> MATLAB Function/1(input1)
  In2/1 -> MATLAB Function/2(input2)
  [LEFTY_MODE] -> MATLAB Function/3(leftyMode)

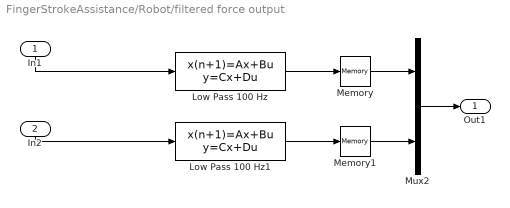
== system FingerStrokeAssistance/Robot/filtered force output ==
  In1 : Inport
  In2 : Inport  Port=2
  Low Pass 100 Hz : DiscreteStateSpace  A=Alow  B=Blow  C=Clow  D=Dlow  X0=x0low  SampleTime=-1
  Low Pass 100 Hz1 : DiscreteStateSpace  A=Alow  B=Blow  C=Clow  D=Dlow  X0=x0low  SampleTime=-1
  Memory : Memory
  Memory1 : Memory
  Mux2 : Mux  Inputs=2
  Out1 : Outport
  wires:
  Low Pass 100 Hz1/1 -> Memory1/1
  Low Pass 100 Hz/1 -> Memory/1
  Mux2/1 -> Out1/1
  In1/1 -> Low Pass 100 Hz/1
  In2/1 -> Low Pass 100 Hz1/1
  Memory/1 -> Mux2/1
  Memory1/1 -> Mux2/2

== system FingerStrokeAssistance/Robot/gravDir ==
  In1 : Inport
  Constant : Constant  Value=1.5
  Sum : Sum  Inputs=|+-
  gain : Gain  Gain=.172
  tag scope: G_ACCEL=global
  wires:
  gain/1 -> [G_ACCEL]
  Sum/1 -> gain/1
  Constant/1 -> Sum/2
  In1/1 -> Sum/1

== system FingerStrokeAssistance/parameters/gain transition ==
  targ : Inport
  Memory : Memory  X0=zeros(1,4)
  gainramp : MATLAB Function  TreatAsAtomicUnit=on
  val : Outport
  wires:
  Memory/1 -> gainramp/3(state)
  gainramp/2(state1) -> Memory/1
  [TRANS_TIME] -> gainramp/1(tr)
  gainramp/1(val) -> val/1
  targ/1 -> gainramp/2(valD)

== system FingerStrokeAssistance/parameters/gain transition1 ==
  targ : Inport
  Memory : Memory  X0=zeros(1,4)
  gainramp : MATLAB Function  TreatAsAtomicUnit=on
  val : Outport
  wires:
  Memory/1 -> gainramp/3(state)
  gainramp/2(state1) -> Memory/1
  [TRANS_TIME] -> gainramp/1(tr)
  gainramp/1(val) -> val/1
  targ/1 -> gainramp/2(valD)

== system FingerStrokeAssistance/parameters/gain transition2 ==
  targ : Inport
  Memory : Memory  X0=zeros(1,4)
  gainramp : MATLAB Function  TreatAsAtomicUnit=on
  val : Outport
  wires:
  Memory/1 -> gainramp/3(state)
  gainramp/2(state1) -> Memory/1
  [TRANS_TIME] -> gainramp/1(tr)
  gainramp/1(val) -> val/1
  targ/1 -> gainramp/2(valD)

== system FingerStrokeAssistance/parameters/gain transition3 ==
  targ : Inport
  Memory : Memory  X0=zeros(1,4)
  gainramp : MATLAB Function  TreatAsAtomicUnit=on
  val : Outport
  wires:
  Memory/1 -> gainramp/3(state)
  gainramp/2(state1) -> Memory/1
  [TRANS_TIME] -> gainramp/1(tr)
  gainramp/1(val) -> val/1
  targ/1 -> gainramp/2(valD)

== system FingerStrokeAssistance/parameters/gain transition4 ==
  targ : Inport
  Memory : Memory  X0=zeros(1,4)
  gainramp : MATLAB Function  TreatAsAtomicUnit=on
  val : Outport
  wires:
  Memory/1 -> gainramp/3(state)
  gainramp/2(state1) -> Memory/1
  [TRANS_TIME] -> gainramp/1(tr)
  gainramp/1(val) -> val/1
  targ/1 -> gainramp/2(valD)

== system FingerStrokeAssistance/parameters/gain transition5 ==
  targ : Inport
  Memory : Memory  X0=zeros(1,4)
  gainramp : MATLAB Function  TreatAsAtomicUnit=on
  val : Outport
  wires:
  Memory/1 -> gainramp/3(state)
  gainramp/2(state1) -> Memory/1
  [TRANS_TIME] -> gainramp/1(tr)
  gainramp/1(val) -> val/1
  targ/1 -> gainramp/2(valD)

== matlab function FingerStrokeAssistance/LL Force Controller/Subsystem/MATLAB Function1 ==
  data: f_ref_pid_2 input; f_ref_pid_1 output; f_ths input; f_spring input; gain input; pos_meas input
function f_ref_pid_1 = fcn(f_ref_pid_2,f_ths,f_spring,gain,pos_meas)
%#codegen

if abs(f_ref_pid_2)>= f_ths
    
    f_ref_pid_1=f_ref_pid_2*gain;
else
    f_ref_pid_1=f_spring*pos_meas(1);
end
end

== matlab function FingerStrokeAssistance/MATLAB Function ==
  data: state input; state output; main_switch input; control_switch input; t_ramp input; k_ramp input; ip_ramp input; f_ref_pid input; f_ref_force input; fp_ramp input; pos_meas input; pos_ref_g input; f_ref output; ramp_switch output; fp_ramp_switch output; f_ref_lim output; enc_trigger output; pos_ref output; pos_ref_Ulim output; pos_ref_Llim output; ff input; f_ths input; f_spring input; gain input; sd_gain input
%% Create Finite State Machine for FINGER Robot

function [state,f_ref,ramp_switch,fp_ramp_switch,f_ref_lim,enc_trigger,pos_ref,pos_ref_Ulim,pos_ref_Llim] = StateMachine(state,main_switch,control_switch,t_ramp,k_ramp,ip_ramp,f_ref_pid,f_ref_force,fp_ramp,pos_meas,pos_ref_g,ff,f_ths,f_spring,gain,sd_gain)
%#codegen

ramp_switch = 0;
fp_ramp_switch = 0;
f_ref = [0 0]';
f_ref_lim = 0;
enc_trigger = 0;
pos_ref_Ulim = 1;
pos_ref_Llim = 0;
pos_ref = pos_meas;

switch state
    
    case 1 %standby phase
        f_ref=[0 0]'; % establish reference force
        f_ref_lim=0; % establish limit for reference force
        
        if main_switch==1  % If the main switch is on proceed to next state
            state=2;
        end
        
    case 2 %Move both linkage arms to position zero
        pos_ref_Ulim = inf;
        pos_ref_Llim = -inf;
        pos_ref = pos_meas;
        ramp_switch = 1; % Define value of ramp switch
        f_ref=[t_ramp*k_ramp t_ramp*k_ramp]'; % Calculate reference force
        f_ref_lim=2.5; % re-establish limit for reference force
        
        if (t_ramp >= 10)
            enc_trigger = 1;  %Calibrate Encoders
            ramp_switch = 0;
            state = 3;
        end
        
    case 3 %Move second finger to flex position
        fp_ramp_switch = 1;
        pos_ref = [0 fp_ramp*ip_ramp]';
        pos_ref_Ulim = 1;
        pos_ref_Llim = 0;
        
     if control_switch == 1
        f_ref = f_ref_force; 
        f_ref_lim = 2.5; 
       else
        f_ref = f_ref_pid; 
        f_ref_lim = 2.5; 
     end

        if (pos_meas(2)>=.9) && (control_switch == 1)
            fp_ramp_switch = 0;
            state = 5;
        elseif (pos_meas(2)>= .9) && (control_switch == 0)
            fp_ramp_switch = 0; 
            state = 4; 
        else
            state = 3;
        end
        
    case 4  %Operating Mode_Position Control - Control first finger linkage
        pos_ref = [pos_ref_g 0.9]';
        f_ref= f_ref_pid;
        pos_ref_Ulim = 1;
        pos_ref_Llim = 0;
        f_ref_lim = 5;   
        
        if main_switch == 0 
            state = 1; 
        end
        
 case 5
             pos_ref = [pos_ref_g 0.9]';
             pos_ref_Ulim = 1;
             pos_ref_Llim = 0;
             f_ref_lim = 2.5;
             
             if f_ref_force(2)>0
                 ff=ff;
             else
                 ff=-ff;
             end
             
             if abs(f_ref_force(2))>= f_ths
                 
                 f_ref_force(1)=f_ref_force(2)*gain;
             else
                 f_ref_force(1)=f_spring*pos_meas(1);
             end 
             
%              if pos_meas(1) >= .9
%                  f_ref_force(1) = f_ref_force(2)*sd_gain; 
%              end
             
              f_ref = [f_ref_force(1) f_ref_force(2)]';
             if main_switch == 0
                 state = 1;
             end


        
end
end

== matlab function FingerStrokeAssistance/LL Force Controller/Subsystem/MATLAB Function2 ==
  data: f_ref_pid_2 input; ff output; ff input
function ff = fcn(f_ref_pid_2,ff)
%#codegen

if f_ref_pid_2>0
    ff=ff;
else
    ff=-ff;
end

end

== matlab function FingerStrokeAssistance/Robot/account for handedness/MATLAB Function ==
  data: input1 input; output1 output; input2 input; leftyMode input; output2 output
% encoder 1 and output 1 relate to the blue mechanism
% encoder 2, output 2 and accel 2 relate to the gold mechanism
% in right hand mode, we want the gold mechanism to control the index finger
% in left hand mode, we want the blue mechanism to control the index finger

% we wallways want the index finger to be finger 1

function [output1, output2] = fcn(input1, input2, leftyMode)
%#codegen
if leftyMode == 1
    output1 = input1;
    output2 = input2;
else
    output1 = input2;
    output2 = input1;
end

== matlab function FingerStrokeAssistance/Robot/account for handedness1/MATLAB Function ==
  data: input1 input; output1 output; input2 input; leftyMode input; output2 output
% encoder 1 and output 1 relate to the blue mechanism
% encoder 2, output 2 and accel 2 relate to the gold mechanism
% in right hand mode, we want the gold mechanism to control the index finger
% in left hand mode, we want the blue mechanism to control the index finger

% we wallways want the index finger to be finger 1

function [output1, output2] = fcn(input1, input2, leftyMode)
%#codegen
if leftyMode == 1
    output1 = input1;
    output2 = input2;
else
    output1 = input2;
    output2 = input1;
end

== matlab function FingerStrokeAssistance/Robot/account for handedness2/MATLAB Function ==
  data: input1 input; output1 output; input2 input; leftyMode input; output2 output
% encoder 1 and output 1 relate to the blue mechanism
% encoder 2, output 2 and accel 2 relate to the gold mechanism
% in right hand mode, we want the gold mechanism to control the index finger
% in left hand mode, we want the blue mechanism to control the index finger

% we wallways want the index finger to be finger 1

function [output1, output2] = fcn(input1, input2, leftyMode)
%#codegen
if leftyMode == 1
    output1 = input1;
    output2 = input2;
else
    output1 = input2;
    output2 = input1;
end

== matlab function FingerStrokeAssistance/parameters/gain transition/gainramp ==
  data: val output; tr input; valD input; state1 output; state input
% state contains [valD_,val_,Ro_,t_]
function [val,state1] = fcn(tr,valD,state)
%#eml

% first we need to check if they have changed the desired Value
if ~ (valD == state(1))
    state(1) = valD;
    state(4) = 0;
    state(3) = state(1) - state(2);
end

t = state(4);
Ro = state(3);

if ((t <= tr) && (tr~=0))
    Rd = Ro - Ro*(10*(t)^3/(tr)^3 - 15*(t)^4/(tr)^4 + 6*(t)^5/(tr)^5);
else
    Rd = 0;
end

val = state(1) - Rd;
state(2) = val;
state(4) = t + .001;
state1 = state;

== matlab function FingerStrokeAssistance/parameters/gain transition1/gainramp ==
  data: val output; tr input; valD input; state1 output; state input
% state contains [valD_,val_,Ro_,t_]
function [val,state1] = fcn(tr,valD,state)
%#eml

% first we need to check if they have changed the desired Value
if ~ (valD == state(1))
    state(1) = valD;
    state(4) = 0;
    state(3) = state(1) - state(2);
end

t = state(4);
Ro = state(3);

if ((t <= tr) && (tr~=0))
    Rd = Ro - Ro*(10*(t)^3/(tr)^3 - 15*(t)^4/(tr)^4 + 6*(t)^5/(tr)^5);
else
    Rd = 0;
end

val = state(1) - Rd;
state(2) = val;
state(4) = t + .001;
state1 = state;

== matlab function FingerStrokeAssistance/parameters/gain transition2/gainramp ==
  data: val output; tr input; valD input; state1 output; state input
% state contains [valD_,val_,Ro_,t_]
function [val,state1] = fcn(tr,valD,state)
%#eml

% first we need to check if they have changed the desired Value
if ~ (valD == state(1))
    state(1) = valD;
    state(4) = 0;
    state(3) = state(1) - state(2);
end

t = state(4);
Ro = state(3);

if ((t <= tr) && (tr~=0))
    Rd = Ro - Ro*(10*(t)^3/(tr)^3 - 15*(t)^4/(tr)^4 + 6*(t)^5/(tr)^5);
else
    Rd = 0;
end

val = state(1) - Rd;
state(2) = val;
state(4) = t + .001;
state1 = state;

== matlab function FingerStrokeAssistance/parameters/gain transition3/gainramp ==
  data: val output; tr input; valD input; state1 output; state input
% state contains [valD_,val_,Ro_,t_]
function [val,state1] = fcn(tr,valD,state)
%#eml

% first we need to check if they have changed the desired Value
if ~ (valD == state(1))
    state(1) = valD;
    state(4) = 0;
    state(3) = state(1) - state(2);
end

t = state(4);
Ro = state(3);

if ((t <= tr) && (tr~=0))
    Rd = Ro - Ro*(10*(t)^3/(tr)^3 - 15*(t)^4/(tr)^4 + 6*(t)^5/(tr)^5);
else
    Rd = 0;
end

val = state(1) - Rd;
state(2) = val;
state(4) = t + .001;
state1 = state;

== matlab function FingerStrokeAssistance/Robot/account for handedness force/MATLAB Function ==
  data: inp1 input; output output; leftyMode input
% channel1 - gold tip
% channel2 - blue tip
% channel3 - gold base
% channel4 - blue base
% we wallways want the index finger to be finger 1

function output = fcn(inp1, leftyMode)
%#codegen

if leftyMode == 1
    output = [inp1(4); inp1(2); inp1(3); inp1(1); inp1(5)];
else
    output = [inp1(3); inp1(1); inp1(4); inp1(2); inp1(5)];
    %output = [inp1(3,1); inp1(4,2); inp1(5)];
end

== matlab function FingerStrokeAssistance/parameters/gain transition4/gainramp ==
  data: val output; tr input; valD input; state1 output; state input
% state contains [valD_,val_,Ro_,t_]
function [val,state1] = fcn(tr,valD,state)
%#eml

% first we need to check if they have changed the desired Value
if ~ (valD == state(1))
    state(1) = valD;
    state(4) = 0;
    state(3) = state(1) - state(2);
end

t = state(4);
Ro = state(3);

if ((t <= tr) && (tr~=0))
    Rd = Ro - Ro*(10*(t)^3/(tr)^3 - 15*(t)^4/(tr)^4 + 6*(t)^5/(tr)^5);
else
    Rd = 0;
end

val = state(1) - Rd;
state(2) = val;
state(4) = t + .001;
state1 = state;

== matlab function FingerStrokeAssistance/parameters/gain transition5/gainramp ==
  data: val output; tr input; valD input; state1 output; state input
% state contains [valD_,val_,Ro_,t_]
function [val,state1] = fcn(tr,valD,state)
%#eml

% first we need to check if they have changed the desired Value
if ~ (valD == state(1))
    state(1) = valD;
    state(4) = 0;
    state(3) = state(1) - state(2);
end

t = state(4);
Ro = state(3);

if ((t <= tr) && (tr~=0))
    Rd = Ro - Ro*(10*(t)^3/(tr)^3 - 15*(t)^4/(tr)^4 + 6*(t)^5/(tr)^5);
else
    Rd = 0;
end

val = state(1) - Rd;
state(2) = val;
state(4) = t + .001;
state1 = state;
